simulink model "ESE4481LController"  (R2024a)
settings: Solver=VariableStepAuto  StartTime=0.0  StopTime=10.0  RelTol=1e-3
undefined symbols (not defined in the file): g, Jx, Kp, Kpe, Kphi, Kv, Pec
settings Model: Creator=achic  LastModifiedBy=achic

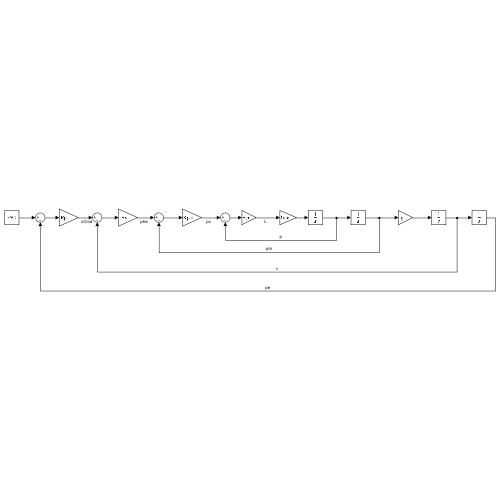
[thumbnail: Simulink's stored preview of the top-level diagram]
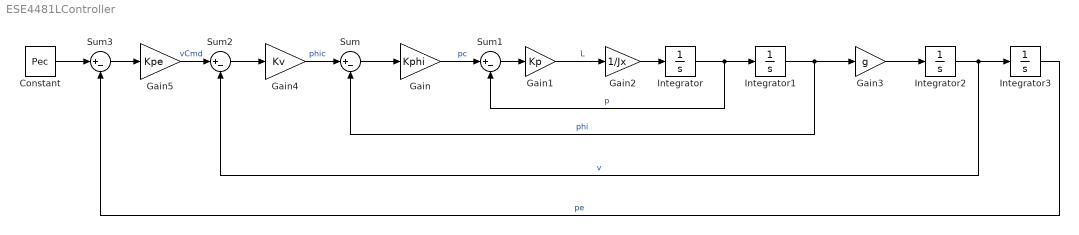
== system ESE4481LController ==
  Constant : Constant  Value=Pec
  Gain : Gain  Gain=Kphi
  Gain1 : Gain  Gain=Kp
  Gain2 : Gain  Gain=1/Jx
  Gain3 : Gain  Gain=g
  Gain4 : Gain  Gain=Kv
  Gain5 : Gain  Gain=Kpe
  Integrator{,1..3} (4 alike) : Integrator
  Sum{,1..3} (4 alike) : Sum  Inputs=|+-
  wires:
  Gain4/1 -> Sum/1  "phic"
  Gain1/1 -> Gain2/1  "L"
  Integrator1/1 -> Gain3/1, Sum/2  "phi"
  Gain/1 -> Sum1/1  "pc"
  Gain2/1 -> Integrator/1
  Integrator/1 -> Integrator1/1, Sum1/2  "p"
  Gain3/1 -> Integrator2/1
  Integrator2/1 -> Integrator3/1, Sum2/2  "v"
  Gain5/1 -> Sum2/1  "vCmd"
  Integrator3/1 -> Sum3/2  "pe"
  Constant/1 -> Sum3/1
  Sum1/1 -> Gain1/1
  Sum/1 -> Gain/1
  Sum2/1 -> Gain4/1
  Sum3/1 -> Gain5/1
